simulink model "tello"  (R2021a)
settings: Solver=VariableStepAuto  StartTime=0.0  StopTime=10000.0  RelTol=1e-3
libraries: dspnetwork x3, instrumentlib x2, aerolibanimutils x1
settings Model: Creator=l.ribeiro-lustosa  LastModifiedBy=l.ribeiro-lustosa

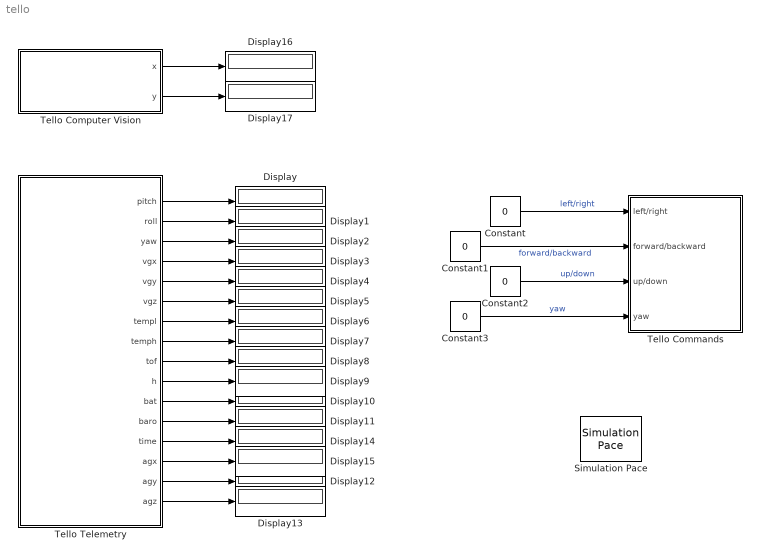
== system tello ==
  Constant : Constant  Value=0  OutDataTypeStr=int32  SampleTime=0.01
  Constant1 : Constant  Value=0  OutDataTypeStr=int32
  Constant2 : Constant  Value=0  OutDataTypeStr=int32
  Constant3 : Constant  Value=0  OutDataTypeStr=int32
  Display{,1..17} (18 alike) : Display
  Simulation Pace : aerolibanimutils/Simulation Pace  SimulationPace=1  SleepMode=Auto  OutputPaceError=off  SampleTime=1/30
  Tello Commands : Subsystem
  Tello Computer Vision : Subsystem
  Tello Telemetry : Subsystem
  wires:
  Constant/1 -> Tello Commands/1(left/right)  "left/right"
  Constant1/1 -> Tello Commands/2(forward/backward)  "forward/backward"
  Constant2/1 -> Tello Commands/3(up/down)  "up/down"
  Constant3/1 -> Tello Commands/4(yaw)  "yaw"
  Tello Telemetry/1(pitch) -> Display/1
  Tello Telemetry/2(roll) -> Display1/1
  Tello Telemetry/3(yaw) -> Display2/1
  Tello Telemetry/4(vgx) -> Display3/1
  Tello Telemetry/5(vgy) -> Display4/1
  Tello Telemetry/6(vgz) -> Display5/1
  Tello Telemetry/7(templ) -> Display6/1
  Tello Telemetry/8(temph) -> Display7/1
  Tello Telemetry/9(tof) -> Display8/1
  Tello Telemetry/10(h) -> Display9/1
  Tello Telemetry/11(bat) -> Display10/1
  Tello Telemetry/12(baro) -> Display11/1
  Tello Telemetry/13(time) -> Display14/1
  Tello Telemetry/14(agx) -> Display15/1
  Tello Telemetry/15(agy) -> Display12/1
  Tello Telemetry/16(agz) -> Display13/1
  Tello Computer Vision/1(x) -> Display16/1
  Tello Computer Vision/2(y) -> Display17/1

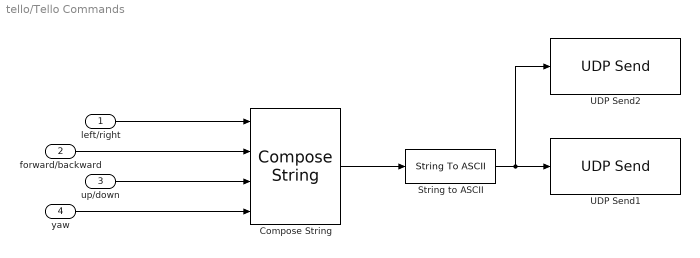
== system tello/Tello Commands ==
  left/right : Inport
  forward/backward : Inport  Port=2
  up/down : Inport  Port=3
  yaw : Inport  Port=4
  Compose String : ComposeString  Format="\"rc %d %d %d %d\""
  String to ASCII : StringToASCII
  UDP Send1 : instrumentlib/UDP Send  Host=127.0.0.1  Port=8889  LocalPort=-1  EnablePortSharing=off  ByteOrder=BigEndian  OutputDatagramPacketSize=512  EnableBlockingMode=on  LocalAddress=0.0.0.0
  UDP Send2 : instrumentlib/UDP Send  Host=192.168.10.1  Port=8889  LocalPort=-1  EnablePortSharing=off  ByteOrder=BigEndian  OutputDatagramPacketSize=512  EnableBlockingMode=on  LocalAddress=0.0.0.0
  wires:
  Compose String/1 -> String to ASCII/1
  left/right/1 -> Compose String/1
  yaw/1 -> Compose String/4
  up/down/1 -> Compose String/3
  forward/backward/1 -> Compose String/2
  String to ASCII/1 -> UDP Send2/1, UDP Send1/1

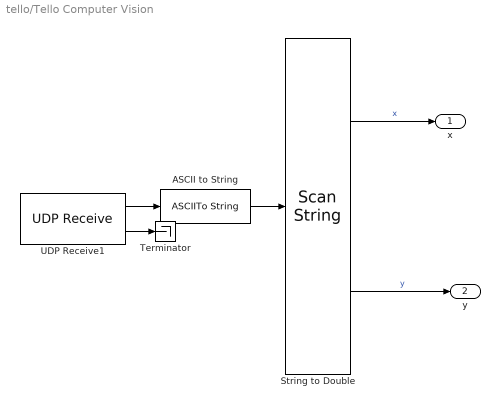
== system tello/Tello Computer Vision ==
  ASCII to String : ASCIIToString
  String to Double : ScanString  Format="\"x:%d;y:%d;\""
  Terminator : Terminator
  UDP Receive1 : dspnetwork/UDP Receive  localURL='0.0.0.0'  localPort=11112  remoteURL='127.0.0.1'  remotePort=-1  recvBufferSize=8192  dims=255  signalDatatype=uint8  isComplex=off  isVarSize=off  showBlockingTime=off  blockingTime=0  sampletime=0.01  blockPlatform=[]
  x : Outport
  y : Outport  Port=2
  wires:
  ASCII to String/1 -> String to Double/1
  UDP Receive1/1 -> ASCII to String/1
  String to Double/2 -> y/1  "y"
  UDP Receive1/2 -> Terminator/1
  String to Double/1 -> x/1  "x"

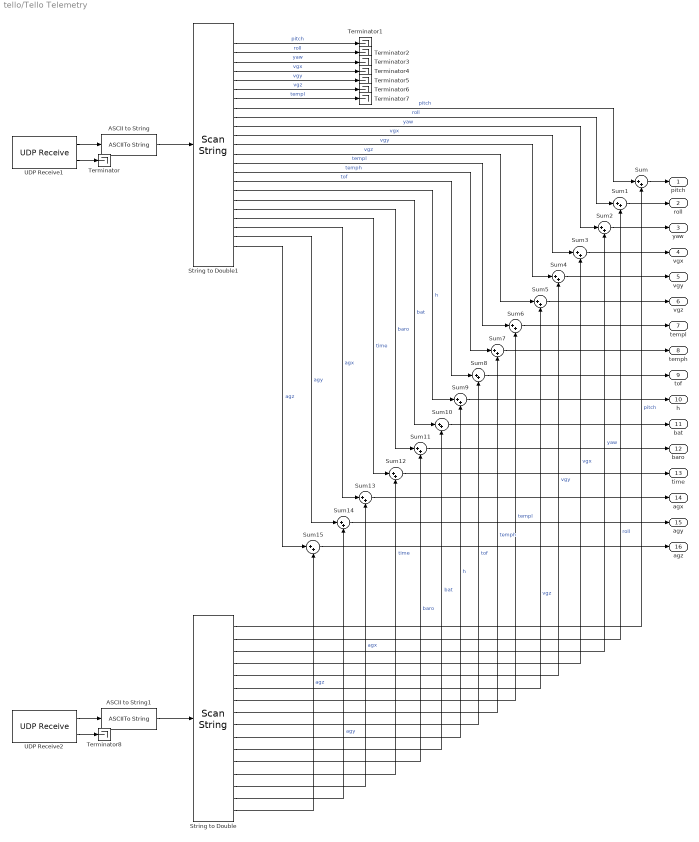
== system tello/Tello Telemetry ==
  ASCII to String : ASCIIToString
  ASCII to String1 : ASCIIToString
  String to Double : ScanString  Format="\"pitch:%d;roll:%d;yaw:%d;vgx:%d;vgy:%d;vgz:%d;templ:%d;temph:%d;tof:%d;h:%d;bat:%d;baro:%d;time:%d;agx:%f;agy:%f;agz:%f;\""
  String to Double1 : ScanString  Format="\"mid:%d;x:%d;y:%d;z:%d;mpry:%d,%d,%d;pitch:%d;roll:%d;yaw:%d;vgx:%d;vgy:%d;vgz:%d;templ:%d;temph:%d;tof:%d;h:%d;bat:%d;baro:%d;time:%d;agx:%f;agy:%f;agz:%f;\""
  Sum{,1..15} (16 alike) : Sum  Inputs=|++
  Terminator{,1..8} (9 alike) : Terminator
  UDP Receive1 : dspnetwork/UDP Receive  localURL='0.0.0.0'  localPort=8890  remoteURL='192.168.10.1'  remotePort=-1  recvBufferSize=8192  dims=255  signalDatatype=uint8  isComplex=off  isVarSize=off  showBlockingTime=off  blockingTime=0  sampletime=0.01  blockPlatform=[]
  UDP Receive2 : dspnetwork/UDP Receive  localURL='0.0.0.0'  localPort=8890  remoteURL='127.0.0.1'  remotePort=-1  recvBufferSize=8192  dims=255  signalDatatype=uint8  isComplex=off  isVarSize=off  showBlockingTime=off  blockingTime=0  sampletime=0.01  blockPlatform=[]
  pitch : Outport
  roll : Outport  Port=2
  yaw : Outport  Port=3
  vgx : Outport  Port=4
  vgy : Outport  Port=5
  vgz : Outport  Port=6
  templ : Outport  Port=7
  temph : Outport  Port=8
  tof : Outport  Port=9
  h : Outport  Port=10
  bat : Outport  Port=11
  baro : Outport  Port=12
  time : Outport  Port=13
  agx : Outport  Port=14
  agy : Outport  Port=15
  agz : Outport  Port=16
  wires:
  String to Double1/20 -> Sum12/1  "time"
  ASCII to String/1 -> String to Double1/1
  String to Double1/17 -> Sum9/1  "h"
  String to Double1/14 -> Sum6/1  "templ"
  UDP Receive1/1 -> ASCII to String/1
  String to Double1/11 -> Sum3/1  "vgx"
  String to Double1/12 -> Sum4/1  "vgy"
  String to Double1/22 -> Sum14/1  "agy"
  String to Double1/18 -> Sum10/1  "bat"
  String to Double1/15 -> Sum7/1  "temph"
  String to Double1/16 -> Sum8/1  "tof"
  String to Double1/13 -> Sum5/1  "vgz"
  String to Double1/9 -> Sum1/1  "roll"
  String to Double1/21 -> Sum13/1  "agx"
  String to Double1/19 -> Sum11/1  "baro"
  String to Double1/23 -> Sum15/1  "agz"
  UDP Receive1/2 -> Terminator/1
  String to Double1/10 -> Sum2/1  "yaw"
  String to Double1/8 -> Sum/1  "pitch"
  String to Double1/1 -> Terminator1/1  "pitch"
  String to Double1/2 -> Terminator2/1  "roll"
  String to Double1/3 -> Terminator3/1  "yaw"
  String to Double1/4 -> Terminator4/1  "vgx"
  String to Double1/5 -> Terminator5/1  "vgy"
  String to Double1/6 -> Terminator6/1  "vgz"
  String to Double1/7 -> Terminator7/1  "templ"
  UDP Receive2/1 -> ASCII to String1/1
  UDP Receive2/2 -> Terminator8/1
  ASCII to String1/1 -> String to Double/1
  Sum/1 -> pitch/1
  String to Double/1 -> Sum/2  "pitch"
  Sum1/1 -> roll/1
  String to Double/2 -> Sum1/2  "roll"
  Sum2/1 -> yaw/1
  String to Double/3 -> Sum2/2  "yaw"
  Sum3/1 -> vgx/1
  String to Double/4 -> Sum3/2  "vgx"
  String to Double/5 -> Sum4/2  "vgy"
  Sum4/1 -> vgy/1
  String to Double/6 -> Sum5/2  "vgz"
  Sum5/1 -> vgz/1
  String to Double/7 -> Sum6/2  "templ"
  Sum6/1 -> templ/1
  Sum7/1 -> temph/1
  String to Double/8 -> Sum7/2  "temph"
  Sum8/1 -> tof/1
  String to Double/9 -> Sum8/2  "tof"
  String to Double/10 -> Sum9/2  "h"
  Sum9/1 -> h/1
  String to Double/11 -> Sum10/2  "bat"
  Sum10/1 -> bat/1
  Sum11/1 -> baro/1
  String to Double/12 -> Sum11/2  "baro"
  Sum12/1 -> time/1
  String to Double/13 -> Sum12/2  "time"
  Sum13/1 -> agx/1
  String to Double/14 -> Sum13/2  "agx"
  Sum14/1 -> agy/1
  String to Double/15 -> Sum14/2  "agy"
  Sum15/1 -> agz/1
  String to Double/16 -> Sum15/2  "agz"
